simulink model "sim3_1_2"  (R2017b)
settings: Solver=ode5  StartTime=0.0  StopTime=20  FixedStep=0.001  RelTol=1e-3
values from neighbouring files (symbols this model uses):
  si = 10    [project.m]
settings Model: Creator=kiran  LastModifiedBy=kiran

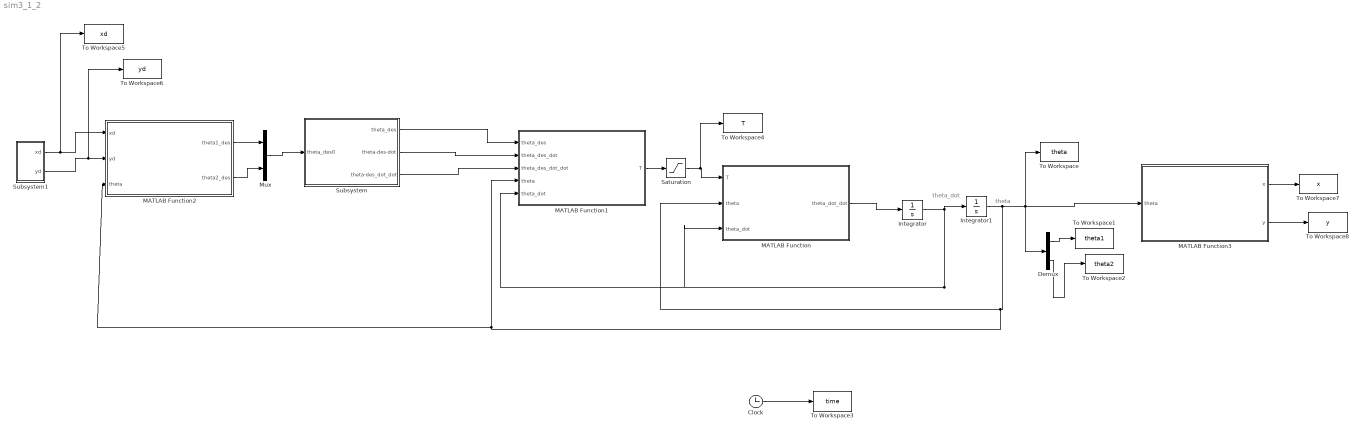
== system sim3_1_2 ==
  note: theta
  note: theta_dot
  Clock : Clock
  Demux : Demux  Outputs=2
  Integrator : Integrator  InitialCondition=[0;0]
  Integrator1 : Integrator  InitialCondition=[-pi/2;0]
  MATLAB Function : MATLAB Function  TreatAsAtomicUnit=on
  MATLAB Function1 : MATLAB Function  TreatAsAtomicUnit=on
  MATLAB Function2 : MATLAB Function  TreatAsAtomicUnit=on
  MATLAB Function3 : MATLAB Function  TreatAsAtomicUnit=on
  Mux : Mux  Inputs=2
  Saturation : Saturate  UpperLimit=5  LowerLimit=-5
  Subsystem : Subsystem
  Subsystem1 : Subsystem
  To Workspace : ToWorkspace  VariableName=theta  SampleTime=-1
  To Workspace1 : ToWorkspace  VariableName=theta1  SampleTime=-1
  To Workspace2 : ToWorkspace  VariableName=theta2  SampleTime=-1
  To Workspace3 : ToWorkspace  VariableName=time  SampleTime=-1
  To Workspace4 : ToWorkspace  VariableName=T  SampleTime=-1
  To Workspace5 : ToWorkspace  VariableName=xd  SampleTime=-1
  To Workspace6 : ToWorkspace  VariableName=yd  SampleTime=-1
  To Workspace7 : ToWorkspace  VariableName=x  SampleTime=-1
  To Workspace8 : ToWorkspace  VariableName=y  SampleTime=-1
  wires:
  MATLAB Function/1(theta_dot_dot) -> Integrator/1
  Integrator/1 -> MATLAB Function1/5(theta_dot), MATLAB Function/3(theta_dot), Integrator1/1
  Integrator1/1 -> MATLAB Function2/3(theta), MATLAB Function1/4(theta), MATLAB Function/2(theta), MATLAB Function3/1(theta), Demux/1, To Workspace/1
  Demux/1 -> To Workspace1/1
  Demux/2 -> To Workspace2/1
  Clock/1 -> To Workspace3/1
  Saturation/1 -> To Workspace4/1, MATLAB Function/1(T)
  MATLAB Function1/1(T) -> Saturation/1
  Subsystem/1(theta_des) -> MATLAB Function1/1(theta_des)
  Subsystem/2(theta-des-dot) -> MATLAB Function1/2(theta_des_dot)
  Subsystem/3(theta-des_dot_dot) -> MATLAB Function1/3(theta_des_dot_dot)
  MATLAB Function2/1(theta1_des) -> Mux/1
  Mux/1 -> Subsystem/1(theta_des0)
  MATLAB Function2/2(theta2_des) -> Mux/2
  Subsystem1/1(xd) -> To Workspace5/1, MATLAB Function2/1(xd)
  Subsystem1/2(yd) -> To Workspace6/1, MATLAB Function2/2(yd)
  MATLAB Function3/1(x) -> To Workspace7/1
  MATLAB Function3/2(y) -> To Workspace8/1

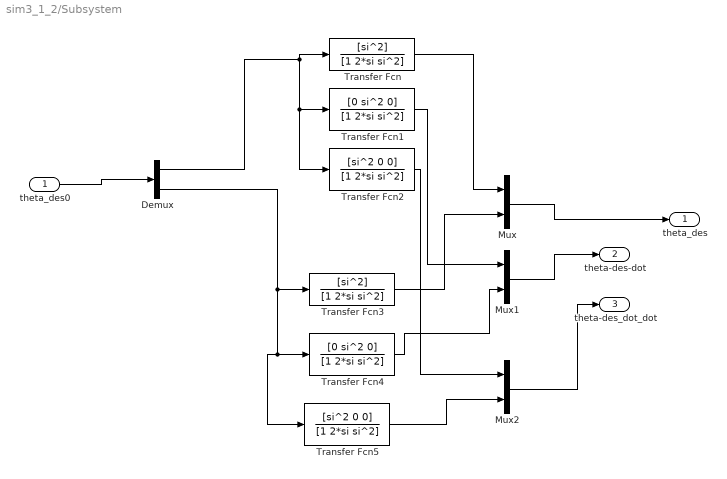
== system sim3_1_2/Subsystem ==
  theta_des0 : Inport
  Demux : Demux  Outputs=2
  Mux : Mux  Inputs=2
  Mux1 : Mux  Inputs=2
  Mux2 : Mux  Inputs=2
  Transfer Fcn : TransferFcn  Numerator=[si^2]  Denominator=[1 2*si si^2]
  Transfer Fcn1 : TransferFcn  Numerator=[0 si^2 0]  Denominator=[1 2*si si^2]
  Transfer Fcn2 : TransferFcn  Numerator=[si^2 0 0]  Denominator=[1 2*si si^2]
  Transfer Fcn3 : TransferFcn  Numerator=[si^2]  Denominator=[1 2*si si^2]
  Transfer Fcn4 : TransferFcn  Numerator=[0 si^2 0]  Denominator=[1 2*si si^2]
  Transfer Fcn5 : TransferFcn  Numerator=[si^2 0 0]  Denominator=[1 2*si si^2]
  theta_des : Outport
  theta-des-dot : Outport  Port=2
  theta-des_dot_dot : Outport  Port=3
  wires:
  Transfer Fcn4/1 -> Mux1/2
  Transfer Fcn5/1 -> Mux2/2
  Transfer Fcn1/1 -> Mux1/1
  Mux/1 -> theta_des/1
  Demux/1 -> Transfer Fcn2/1, Transfer Fcn1/1, Transfer Fcn/1
  Transfer Fcn2/1 -> Mux2/1
  Demux/2 -> Transfer Fcn3/1, Transfer Fcn5/1, Transfer Fcn4/1
  Transfer Fcn/1 -> Mux/1
  Transfer Fcn3/1 -> Mux/2
  Mux2/1 -> theta-des_dot_dot/1
  Mux1/1 -> theta-des-dot/1
  theta_des0/1 -> Demux/1

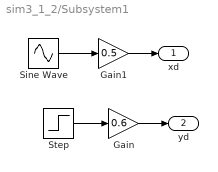
== system sim3_1_2/Subsystem1 ==
  Gain : Gain  Gain=0.6
  Gain1 : Gain  Gain=0.5
  Sine Wave : Sin  SampleTime=0
  Step : Step  Time=0  SampleTime=0
  xd : Outport
  yd : Outport  Port=2
  wires:
  Sine Wave/1 -> Gain1/1
  Gain/1 -> yd/1
  Step/1 -> Gain/1
  Gain1/1 -> xd/1

== matlab function sim3_1_2/MATLAB Function1 ==
  data: theta_des input; theta_des_dot input; theta_des_dot_dot input; T output; theta input; theta_dot input
function T = fcn3(theta_des,theta_des_dot,theta_des_dot_dot, theta, theta_dot)
l1 =0.5;    %m
l2 = 0.3;   %m
r1 = 0.25;  %m
r2 = 0.15;  %m
m1 = 0.5;   %kg
m2 = 0.3;   %kg
I1 = 0.0104;%kg-m^2
I2 = 0.0022;%kg-m^2
c1 = 0;     %N.m.s/rad
c2 = 0;     %N.m.s/rad
g = 9.81;   %m/s^2

alpha = I1+I2+m1*r1^2+m2*(l1^2+r2^2);
beta = m2*l1*r2;
gamma = I2+m2*r2^2;

theta1 = theta(1);
theta2 = theta(2);
theta1_dot = theta_dot(1);
theta2_dot = theta_dot(2);

M =[alpha+2*beta.*cos(theta2) gamma+beta.*cos(theta2); gamma+beta.*cos(theta2) gamma];
C = [c1-beta.*theta2_dot.*sin(theta2) -beta.*(theta1_dot+theta2_dot).*sin(theta2); beta*theta1_dot.*sin(theta2) c2];
N = [(m1*r1+m2*l1)*g.*cos(theta1)+m2*r2*g.*cos(theta1+theta2); m2*r2*g.*cos(theta1+theta2)];


lambda=20;

K1=[2*lambda; 2*lambda];
K2=[lambda^2;lambda^2];

% theta_des1=-3*pi/4;
% theta_des2=pi/4;

e=theta_des-theta;

e_dot=theta_des_dot-theta_dot;

e_dot_dot=-K1.*e_dot-K2.*e;

T=M*theta_des_dot_dot-M*e_dot_dot+C*theta_dot+N;

end

== matlab function sim3_1_2/MATLAB Function ==
  data: T input; theta_dot_dot output; theta input; theta_dot input
function theta_dot_dot = fcn(T,theta,theta_dot)
l1 =0.5;    %m
l2 = 0.3;   %m
r1 = 0.25;  %m
r2 = 0.15;  %m
m1 = 0.48;   %kg
m2 = 0.32;   %kg
I1 = 0.0100;%kg-m^2
I2 = 0.0024;%kg-m^2
c1 = 0;     %N.m.s/rad
c2 = 0;     %N.m.s/rad
g = 9.81;   %m/s^2

alpha = I1+I2+m1*r1^2+m2*(l1^2+r2^2);
beta = m2*l1*r2;
gamma = I2+m2*r2^2;

theta1 = theta(1);
theta2 = theta(2);
theta1_dot = theta_dot(1);
theta2_dot = theta_dot(2);

M =[alpha+2*beta.*cos(theta2) gamma+beta.*cos(theta2); gamma+beta.*cos(theta2) gamma];
C = [c1-beta.*theta2_dot.*sin(theta2) -beta.*(theta1_dot+theta2_dot).*sin(theta2); beta*theta1_dot.*sin(theta2) c2];
N = [(m1*r1+m2*l1)*g.*cos(theta1)+m2*r2*g.*cos(theta1+theta2); m2*r2*g.*cos(theta1+theta2)];

theta_dot_dot = inv(M)*(T-C*theta_dot-N);
end

== matlab function sim3_1_2/MATLAB Function2 ==
  data: xd input; yd input; theta1_des output; theta input; theta2_des output
function [theta1_des,theta2_des]= fcn(xd,yd,theta)
l1 =0.5;    %m
l2 = 0.3;   %m

theta2=theta(2);
theta2_des=acos(((xd^2+yd^2-l1^2-l2^2)/(2*l1*l2)));
theta1_des=atan2(yd,xd)-atan2(l2*sin(theta2),(l1+l2*cos(theta2)));

end

== matlab function sim3_1_2/MATLAB Function3 ==
  data: theta input; x output; y output
function [x,y]= fcn(theta)
l1 =0.5;    %m
l2 = 0.3;   %m
r1 = 0.25;  %m
r2 = 0.15;  %m
m1 = 0.48;   %kg
m2 = 0.32;   %kg
I1 = 0.0100;%kg-m^2
I2 = 0.0024;%kg-m^2
c1 = 0;     %N.m.s/rad
c2 = 0;     %N.m.s/rad
g = 9.81;   %m/s^2

alpha = I1+I2+m1*r1^2+m2*(l1^2+r2^2);
beta = m2*l1*r2;
gamma = I2+m2*r2^2;

theta1 = theta(1);
theta2 = theta(2);

x= l1*cos(theta1)+l2*cos(theta1+theta2);
y= l1*sin(theta1)+l2*sin(theta1+theta2);
end
